simulink model "REFvsFI_ML2017a"  (R2017a)
settings: Solver=FixedStepAuto  StartTime=0.0  StopTime=T  RelTol=1e-3  EnableMultiTasking=on
values from neighbouring files (symbols this model uses):
  Ts = 1    [TestDataGen.m]
libraries: My_FI_Operations x114, simulink x2
(part 1 of 2)
settings Model: FPTShortcutValueString='{{},{''BaselineRun'',1,1,1,''BaselineRun'','''',{},''M'',''D'',''''}}'  OrderedModelArguments=off  Creator=kavru  LastModifiedBy=kolbe
settings DataIOCC: ReturnWorkspaceOutputs=on
settings OptimizationCC: BlockReduction=off  ConditionallyExecuteInputs=off
settings DebuggingCC: SignalRangeChecking=warning  SingleTaskRateTransMsg=error
settings SFSimCC: SimUseLocalCustomCode=on
settings RTWCC: RTWUseLocalCustomCode=on

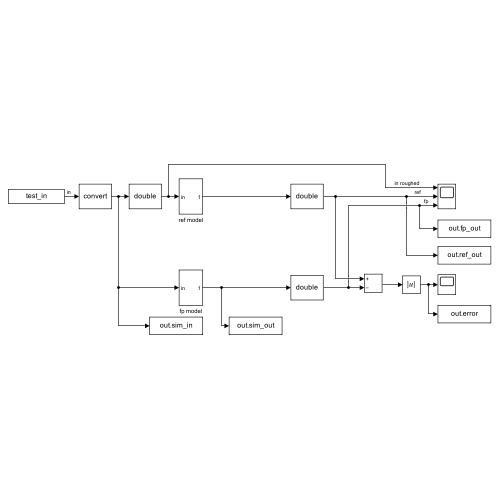
[thumbnail: Simulink's stored preview of the top-level diagram]
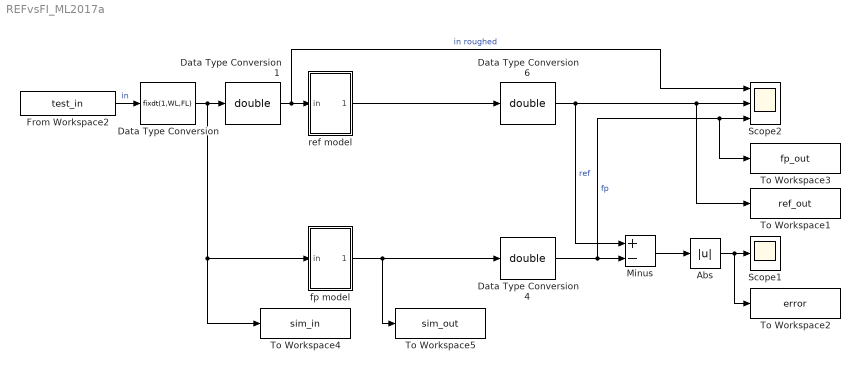
== system REFvsFI_ML2017a ==
  Abs : Abs
  Data Type Conversion : DataTypeConversion  OutDataTypeStr=fixdt(1,WL,FL)  RndMeth=Nearest  SaturateOnIntegerOverflow=on
  Data Type Conversion1 : DataTypeConversion  OutDataTypeStr=double  RndMeth=Nearest
  Data Type Conversion4 : DataTypeConversion  OutDataTypeStr=double  RndMeth=Nearest
  Data Type Conversion6 : DataTypeConversion  OutDataTypeStr=double  RndMeth=Nearest
  From Workspace2 : FromWorkspace  VariableName=test_in  OutDataTypeStr=double  SampleTime=Ts
  Minus : Sum  Inputs=+-
  Scope1 : Scope
  Scope2 : Scope  NumInputPorts=3
  To Workspace1 : ToWorkspace  VariableName=ref_out  SaveFormat=Timeseries  SampleTime=-1
  To Workspace2 : ToWorkspace  VariableName=error  SaveFormat=Timeseries  SampleTime=-1
  To Workspace3 : ToWorkspace  VariableName=fp_out  SaveFormat=Timeseries  SampleTime=-1
  To Workspace4 : ToWorkspace  VariableName=sim_in  SaveFormat=Timeseries  SampleTime=-1
  To Workspace5 : ToWorkspace  VariableName=sim_out  SaveFormat=Timeseries  SampleTime=-1
  fp model : Subsystem
  ref model : Subsystem
  wires:
  From Workspace2/1 -> Data Type Conversion/1  "in"
  Minus/1 -> Abs/1
  Abs/1 -> Scope1/1, To Workspace2/1
  fp model/1(Out1) -> To Workspace5/1, Data Type Conversion4/1
  Data Type Conversion4/1 -> Minus/2, To Workspace3/1, Scope2/3  "fp"
  Data Type Conversion6/1 -> Scope2/2, To Workspace1/1, Minus/1  "ref"
  Data Type Conversion1/1 -> Scope2/1, ref model/1(in)  "in roughed"
  Data Type Conversion/1 -> To Workspace4/1, fp model/1(in), Data Type Conversion1/1
  ref model/1(Out1) -> Data Type Conversion6/1

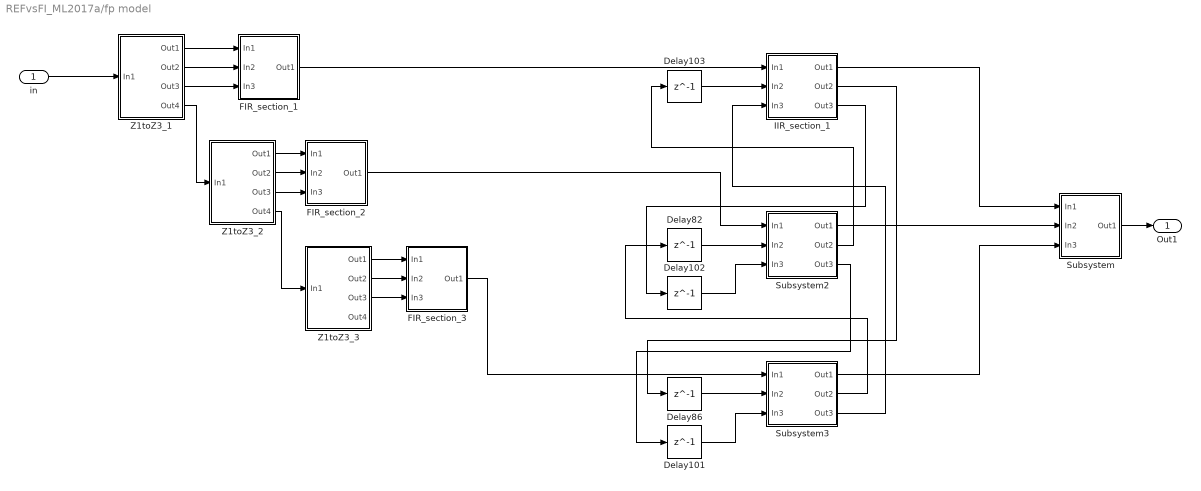
== system REFvsFI_ML2017a/fp model ==
  in : Inport
  Delay{82,86,101..103} (5 alike) : Delay  DelayLength=1  SampleTime=3*Ts
  FIR_section_1 : Subsystem
  FIR_section_2 : Subsystem
  FIR_section_3 : Subsystem
  IIR_section_1 : Subsystem
  Subsystem : Subsystem
  Subsystem2 : Subsystem
  Subsystem3 : Subsystem
  Z1toZ3_1 : Subsystem
  Z1toZ3_2 : Subsystem
  Z1toZ3_3 : Subsystem
  Out1 : Outport
  wires:
  in/1 -> Z1toZ3_1/1(In1)
  Z1toZ3_1/4(Out4) -> Z1toZ3_2/1(In1)
  Z1toZ3_2/4(Out4) -> Z1toZ3_3/1(In1)
  Z1toZ3_1/1(Out1) -> FIR_section_1/1(In1)
  Z1toZ3_1/2(Out2) -> FIR_section_1/2(In2)
  Z1toZ3_1/3(Out3) -> FIR_section_1/3(In3)
  Z1toZ3_2/1(Out1) -> FIR_section_2/1(In1)
  Z1toZ3_2/2(Out2) -> FIR_section_2/2(In2)
  Z1toZ3_2/3(Out3) -> FIR_section_2/3(In3)
  Z1toZ3_3/1(Out1) -> FIR_section_3/1(In1)
  Z1toZ3_3/2(Out2) -> FIR_section_3/2(In2)
  Z1toZ3_3/3(Out3) -> FIR_section_3/3(In3)
  Subsystem/1(Out1) -> Out1/1
  FIR_section_1/1(Out1) -> IIR_section_1/1(In1)
  Delay103/1 -> IIR_section_1/2(In2)
  IIR_section_1/2(Out2) -> Delay86/1
  IIR_section_1/1(Out1) -> Subsystem/1(In1)
  IIR_section_1/3(Out3) -> Delay102/1
  FIR_section_2/1(Out1) -> Subsystem2/1(In1)
  Delay102/1 -> Subsystem2/3(In3)
  Delay82/1 -> Subsystem2/2(In2)
  Subsystem2/1(Out1) -> Subsystem/2(In2)
  Subsystem2/2(Out2) -> Delay103/1
  Subsystem2/3(Out3) -> Delay101/1
  Delay86/1 -> Subsystem3/2(In2)
  Delay101/1 -> Subsystem3/3(In3)
  FIR_section_3/1(Out1) -> Subsystem3/1(In1)
  Subsystem3/3(Out3) -> IIR_section_1/3(In3)
  Subsystem3/1(Out1) -> Subsystem/3(In3)
  Subsystem3/2(Out2) -> Delay82/1

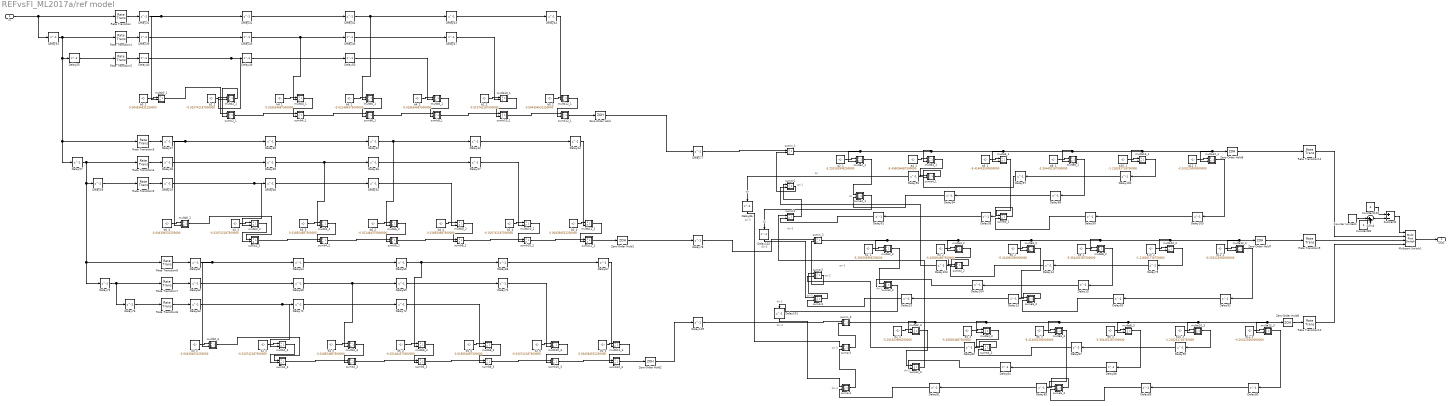
== system REFvsFI_ML2017a/ref model ==
  note: dn-1
  note: dn-2
  note: qn-3
  note: dn-3
  note: qn
  note: dn
  note: dn-4
  note: dn-2
  note: dn-1
  note: qn
  note: dn-4
  note: dn
  note: dn-3
  note: qn-2
  note: qn-3
  note: qn-1
  note: qn-1
  in : Inport
  Constant102 : Constant  Value=4
  Constant82 : Constant
  Counter Limited1 : simulink/Sources/Counter Limited  uplimit=2  tsamp=Ts
  Delay{13..15,23,27..37,39..50,52,60..72,75,77..78,80..82,84..95,97..105,109} (69 alike) : Delay  DelayLength=1  SampleTime=3*Ts
  Delay{53,55,57,59,74,76} (6 alike) : Delay  DelayLength=1  SampleTime=Ts
  Multiport Switch1 : MultiPortSwitch  OutDataTypeStr=double  RndMeth=Nearest
  Rate Transition{,1..8} (9 alike) : RateTransition  OutPortSampleTime=3*Ts
  Rate Transition10 : RateTransition  OutPortSampleTime=Ts
  Rate Transition12 : RateTransition  OutPortSampleTime=Ts
  Rate Transition9 : RateTransition  OutPortSampleTime=Ts
  Subtract2 : Sum  Inputs=+-
  Sum4 : Sum  Inputs=|++
  Zero-Order Hold{,1..2,6..8} (6 alike) : ZeroOrderHold  SampleTime=3*Ts
  a10_1 : Constant  Value=-1.218261718750000  OutDataTypeStr=double
  a10_2 : Constant  Value=-1.218261718750000  OutDataTypeStr=double
  a10_3 : Constant  Value=-1.218261718750000  OutDataTypeStr=double
  a12_1 : Constant  Value=-0.203125000000000  OutDataTypeStr=double
  a12_2 : Constant  Value=-0.203125000000000  OutDataTypeStr=double
  a12_3 : Constant  Value=-0.203125000000000  OutDataTypeStr=double
  a2_1 : Constant  Value=-3.291503906250000  OutDataTypeStr=double
  a2_2 : Constant  Value=-3.291503906250000  OutDataTypeStr=double
  a2_3 : Constant  Value=-3.291503906250000  OutDataTypeStr=double
  a4_1 : Constant  Value=-5.456054687500000  OutDataTypeStr=double
  a4_2 : Constant  Value=-5.456054687500000  OutDataTypeStr=double
  a4_3 : Constant  Value=-5.456054687500000  OutDataTypeStr=double
  a6_1 : Constant  Value=-5.414062500000000  OutDataTypeStr=double
  a6_2 : Constant  Value=-5.414062500000000  OutDataTypeStr=double
  a6_3 : Constant  Value=-5.414062500000000  OutDataTypeStr=double
  a8_1 : Constant  Value=-3.354492187500000  OutDataTypeStr=double
  a8_2 : Constant  Value=-3.354492187500000  OutDataTypeStr=double
  a8_3 : Constant  Value=-3.354492187500000  OutDataTypeStr=double
  b0_{1..6} (6 alike) : Constant  Value=0.004394531250000  OutDataTypeStr=double
  b2_{1..6} (6 alike) : Constant  Value=-0.010742187500000  OutDataTypeStr=double
  b4_{1..6} (6 alike) : Constant  Value=0.018554687500000  OutDataTypeStr=double
  b6_1 : Constant  Value=-0.021484375000000  OutDataTypeStr=double
  b6_2 : Constant  Value=-0.021484375000000  OutDataTypeStr=double
  b6_3 : Constant  Value=-0.021484375000000  OutDataTypeStr=double
  multa10_1 : Subsystem  AncestorBlock=My_FI_Operations/multa10_
      mask Display: disp('x')
  multa10_2 : Subsystem  AncestorBlock=My_FI_Operations/multa10_
      mask Display: disp('x')
  multa10_3 : Subsystem  AncestorBlock=My_FI_Operations/multa10_
      mask Display: disp('x')
  multa12_1 : Subsystem  AncestorBlock=My_FI_Operations/multa12_
      mask Display: disp('x')
  multa12_2 : Subsystem  AncestorBlock=My_FI_Operations/multa12_
      mask Display: disp('x')
  multa12_3 : Subsystem  AncestorBlock=My_FI_Operations/multa12_
      mask Display: disp('x')
  multa2_1 : Subsystem  AncestorBlock=My_FI_Operations/multa2_
      mask Display: disp('x')
  multa2_2 : Subsystem  AncestorBlock=My_FI_Operations/multa2_
      mask Display: disp('x')
  multa2_3 : Subsystem  AncestorBlock=My_FI_Operations/multa2_
      mask Display: disp('x')
  multa4_1 : Subsystem  AncestorBlock=My_FI_Operations/multa4_
      mask Display: disp('x')
  multa4_2 : Subsystem  AncestorBlock=My_FI_Operations/multa4_
      mask Display: disp('x')
  multa4_3 : Subsystem  AncestorBlock=My_FI_Operations/multa4_
      mask Display: disp('x')
  multa6_1 : Subsystem  AncestorBlock=My_FI_Operations/multa6_
      mask Display: disp('x')
  multa6_2 : Subsystem  AncestorBlock=My_FI_Operations/multa6_
      mask Display: disp('x')
  multa6_3 : Subsystem  AncestorBlock=My_FI_Operations/multa6_
      mask Display: disp('x')
  multa8_1 : Subsystem  AncestorBlock=My_FI_Operations/multa8_
      mask Display: disp('x')
  multa8_2 : Subsystem  AncestorBlock=My_FI_Operations/multa8_
      mask Display: disp('x')
  multa8_3 : Subsystem  AncestorBlock=My_FI_Operations/multa8_
      mask Display: disp('x')
  multb0_1 : Subsystem  AncestorBlock=My_FI_Operations/multb0_
      mask Display: disp('x')
  multb0_2 : Subsystem  AncestorBlock=My_FI_Operations/multb0_
      mask Display: disp('x')
  multb0_3 : Subsystem  AncestorBlock=My_FI_Operations/multb0_
      mask Display: disp('x')
  multb10_1 : Subsystem  AncestorBlock=My_FI_Operations/multb10_
      mask Display: disp('x')
  multb10_2 : Subsystem  AncestorBlock=My_FI_Operations/multb10_
      mask Display: disp('x')
  multb10_3 : Subsystem  AncestorBlock=My_FI_Operations/multb10_
      mask Display: disp('x')
  multb12_1 : Subsystem  AncestorBlock=My_FI_Operations/multb12_
      mask Display: disp('x')
  multb12_2 : Subsystem  AncestorBlock=My_FI_Operations/multb12_
      mask Display: disp('x')
  multb12_3 : Subsystem  AncestorBlock=My_FI_Operations/multb12_
      mask Display: disp('x')
  multb2_1 : Subsystem  AncestorBlock=My_FI_Operations/multb2_
      mask Display: disp('x')
  multb2_2 : Subsystem  AncestorBlock=My_FI_Operations/multb2_
      mask Display: disp('x')
  multb2_3 : Subsystem  AncestorBlock=My_FI_Operations/multb2_
      mask Display: disp('x')
  multb4_1 : Subsystem  AncestorBlock=My_FI_Operations/multb4_
      mask Display: disp('x')
  multb4_2 : Subsystem  AncestorBlock=My_FI_Operations/multb4_
      mask Display: disp('x')
  multb4_3 : Subsystem  AncestorBlock=My_FI_Operations/multb4_
      mask Display: disp('x')
  multb6_1 : Subsystem  AncestorBlock=My_FI_Operations/multb6_
      mask Display: disp('x')
  multb6_2 : Subsystem  AncestorBlock=My_FI_Operations/multb6_
      mask Display: disp('x')
  multb6_3 : Subsystem  AncestorBlock=My_FI_Operations/multb6_
      mask Display: disp('x')
  multb8_1 : Subsystem  AncestorBlock=My_FI_Operations/multb8_
      mask Display: disp('x')
  multb8_2 : Subsystem  AncestorBlock=My_FI_Operations/multb8_
      mask Display: disp('x')
  multb8_3 : Subsystem  AncestorBlock=My_FI_Operations/multb8_
      mask Display: disp('x')
  suma2_1 : Subsystem  AncestorBlock=My_FI_Operations/suma2_
      mask Display: disp('+')
  suma2_2 : Subsystem  AncestorBlock=My_FI_Operations/suma2_
      mask Display: disp('+')
  suma2_3 : Subsystem  AncestorBlock=My_FI_Operations/suma2_
      mask Display: disp('+')
  suma4_1 : Subsystem  AncestorBlock=My_FI_Operations/suma4_
      mask Display: disp('+')
  suma4_2 : Subsystem  AncestorBlock=My_FI_Operations/suma4_
      mask Display: disp('+')
  suma4_3 : Subsystem  AncestorBlock=My_FI_Operations/suma4_
      mask Display: disp('+')
  suma6_1 : Subsystem  AncestorBlock=My_FI_Operations/suma6_
      mask Display: disp('+')
  suma6_2 : Subsystem  AncestorBlock=My_FI_Operations/suma6_
      mask Display: disp('+')
  suma6_3 : Subsystem  AncestorBlock=My_FI_Operations/suma6_
      mask Display: disp('+')
  sumb10_1 : Subsystem  AncestorBlock=My_FI_Operations/sumb10_
      mask Display: disp('+')
  sumb10_2 : Subsystem  AncestorBlock=My_FI_Operations/sumb10_
      mask Display: disp('+')
  sumb10_3 : Subsystem  AncestorBlock=My_FI_Operations/sumb10_
      mask Display: disp('+')
  sumb12_1 : Subsystem  AncestorBlock=My_FI_Operations/sumb12_
      mask Display: disp('+')
  sumb12_2 : Subsystem  AncestorBlock=My_FI_Operations/sumb12_
      mask Display: disp('+')
  sumb12_3 : Subsystem  AncestorBlock=My_FI_Operations/sumb12_
      mask Display: disp('+')
  sumb2_1 : Subsystem  AncestorBlock=My_FI_Operations/sumb2_
      mask Display: disp('+')
  sumb2_2 : Subsystem  AncestorBlock=My_FI_Operations/sumb2_
      mask Display: disp('+')
  sumb2_3 : Subsystem  AncestorBlock=My_FI_Operations/sumb2_
      mask Display: disp('+')
  sumb4_1 : Subsystem  AncestorBlock=My_FI_Operations/sumb4_
      mask Display: disp('+')
  sumb4_2 : Subsystem  AncestorBlock=My_FI_Operations/sumb4_
      mask Display: disp('+')
  sumb4_3 : Subsystem  AncestorBlock=My_FI_Operations/sumb4_
      mask Display: disp('+')
  sumb6_1 : Subsystem  AncestorBlock=My_FI_Operations/sumb6_
      mask Display: disp('+')
  sumb6_2 : Subsystem  AncestorBlock=My_FI_Operations/sumb6_
      mask Display: disp('+')
  sumb6_3 : Subsystem  AncestorBlock=My_FI_Operations/sumb6_
      mask Display: disp('+')
  sumb8_1 : Subsystem  AncestorBlock=My_FI_Operations/sumb8_
      mask Display: disp('+')
  sumb8_2 : Subsystem  AncestorBlock=My_FI_Operations/sumb8_
      mask Display: disp('+')
  sumb8_3 : Subsystem  AncestorBlock=My_FI_Operations/sumb8_
      mask Display: disp('+')
  sumd-2 : Subsystem  AncestorBlock=My_FI_Operations/sumd-2
      mask Display: disp('+')
  sumd-3 : Subsystem  AncestorBlock=My_FI_Operations/sumd-3
      mask Display: disp('+')
  sumd-4 : Subsystem  AncestorBlock=My_FI_Operations/sumd-4
      mask Display: disp('+')
  sumin_1 : Subsystem  AncestorBlock=My_FI_Operations/sumin_
      mask Display: disp('+')
  sumin_2 : Subsystem  AncestorBlock=My_FI_Operations/sumin_
      mask Display: disp('+')
  sumin_3 : Subsystem  AncestorBlock=My_FI_Operations/sumin_
      mask Display: disp('+')
  sumq-1 : Subsystem  AncestorBlock=My_FI_Operations/sumq-1
      mask Display: disp('+')
  sumq-2 : Subsystem  AncestorBlock=My_FI_Operations/sumq-2
      mask Display: disp('+')
  sumq-3 : Subsystem  AncestorBlock=My_FI_Operations/sumq-3
      mask Display: disp('+')
  Out1 : Outport
  wires:
  Delay77/1 -> sumin_1/1(In1)
  Delay42/1 -> multb6_1/2(In1), Delay43/1
  multb6_2/1(Out1) -> sumb6_2/2(In1)
  Delay53/1 -> Rate Transition1/1, Rate Transition3/1, Delay57/1, Delay55/1
  Delay78/1 -> sumin_2/1(In1)
  sumin_2/1(Out1) -> multa2_2/2(In1), multa4_2/2(In1), multa6_2/2(In1), multa8_2/2(In1), multa10_2/2(In1), multa12_2/2(In1), Zero-Order Hold7/1
  b0_6/1 -> multb12_3/1(In2)
  Delay69/1 -> Delay70/1
  Delay101/1 -> sumd-4/1(In1)
  Delay31/1 -> multb0_1/2(In1), Delay41/1
  sumq-2/1(Out1) -> sumin_2/2(In2)
  Delay32/1 -> multb6_2/2(In1), Delay33/1
  multa8_3/1(Out1) -> Delay88/1
  multb6_1/1(Out1) -> sumb6_1/2(In1)
  Delay94/1 -> suma2_1/2(In1)
  Delay68/1 -> multb4_3/2(In1), Delay69/1
  Delay41/1 -> Delay42/1
  Delay85/1 -> Delay81/1
  Zero-Order Hold/1 -> Delay77/1
  Delay64/1 -> Delay65/1
  b2_4/1 -> multb10_2/1(In2)
  sumin_1/1(Out1) -> multa2_1/2(In1), multa4_1/2(In1), multa6_1/2(In1), multa8_1/2(In1), multa10_1/2(In1), multa12_1/2(In1), Zero-Order Hold6/1
  sumb4_3/1(Out1) -> sumb6_3/1(In2)
  b4_5/1 -> multb4_3/1(In2)
  Zero-Order Hold2/1 -> Delay109/1
  Zero-Order Hold1/1 -> Delay78/1
  Delay84/1 -> suma2_3/2(In1)
  Delay27/1 -> multb0_2/2(In1), Delay30/1
  in/1 -> Delay53/1, Rate Transition/1
  Delay100/1 -> Delay97/1
  multa2_3/1(Out1) -> suma2_3/1(In2)
  Delay65/1 -> multb6_3/2(In1), Delay66/1
  Delay28/1 -> Delay35/1
  Delay33/1 -> Delay34/1
  Delay57/1 -> Rate Transition4/1, Rate Transition6/1, Delay74/1, Delay59/1
  Delay48/1 -> Delay52/1
  Delay98/1 -> Delay94/1
  multa10_2/1(Out1) -> Delay75/1
  Delay40/1 -> multb2_1/2(In1), Delay49/1
  Delay13/1 -> Delay23/1
  a10_2/1 -> multa10_2/1(In2)
  sumb2_3/1(Out1) -> sumb4_3/1(In2)
  a4_3/1 -> multa4_3/1(In2)
  sumd-3/1(Out1) -> sumq-2/1(In1)
  suma6_3/1(Out1) -> Delay85/1
  sumb12_1/1(Out1) -> Zero-Order Hold/1
  Delay63/1 -> multb2_3/2(In1), Delay71/1
  Multiport Switch1/1 -> Out1/1
  a12_1/1 -> multa12_1/1(In2)
  multb4_3/1(Out1) -> sumb4_3/2(In1)
  multa8_2/1(Out1) -> Delay15/1
  sumq-3/1(Out1) -> sumin_3/2(In2)
  Constant82/1 -> Sum4/2
  Delay15/1 -> Delay104/1
  Delay109/1 -> sumin_3/1(In1)
  Delay86/1 -> sumq-3/1(In1)
  multa4_2/1(Out1) -> suma4_2/1(In1)
  sumd-4/1(Out1) -> sumq-3/2(In2)
  b0_1/1 -> multb0_1/1(In2)
  Delay88/1 -> Delay84/1
  multa6_3/1(Out1) -> suma6_3/1(In1)
  Counter Limited1/1 -> Sum4/1
  sumb6_2/1(Out1) -> sumb8_2/1(In2)
  sumb8_3/1(Out1) -> sumb10_3/1(In2)
  Delay61/1 -> multb0_3/2(In1), Delay64/1
  Delay91/1 -> sumd-2/2(In2)
  multa4_3/1(Out1) -> suma4_3/1(In1)
  a2_3/1 -> multa2_3/1(In2)
  a10_3/1 -> multa10_3/1(In2)
  a12_3/1 -> multa12_3/1(In2)
  b0_2/1 -> multb12_1/1(In2)
  a12_2/1 -> multa12_2/1(In2)
  Delay95/1 -> Delay91/1
  multb12_1/1(Out1) -> sumb12_1/2(In1)
  b2_2/1 -> multb10_1/1(In2)
  a6_3/1 -> multa6_3/1(In2)
  sumin_3/1(Out1) -> multa2_3/2(In1), multa4_3/2(In1), multa6_3/2(In1), multa8_3/2(In1), multa10_3/2(In1), multa12_3/2(In1), Zero-Order Hold8/1
  Delay62/1 -> Delay68/1
  Delay70/1 -> multb10_3/2(In1)
  a4_1/1 -> multa4_1/1(In2)
  Delay74/1 -> Rate Transition7/1, Delay76/1
  Delay50/1 -> multb8_1/2(In1)
  sumd-2/1(Out1) -> sumq-1/1(In2)
  a2_1/1 -> multa2_1/1(In2)
  sumb8_1/1(Out1) -> sumb10_1/1(In2)
  Delay14/1 -> suma4_2/2(In2)
  Delay87/1 -> suma4_3/2(In2)
  a4_2/1 -> multa4_2/1(In2)
  Zero-Order Hold6/1 -> Rate Transition12/1
  Subtract2/1 -> Multiport Switch1/1
  a6_2/1 -> multa6_2/1(In2)
  multb2_3/1(Out1) -> sumb2_3/2(In1)
  multb4_1/1(Out1) -> sumb4_1/2(In1)
  Delay81/1 -> sumd-4/2(In2)
  Delay89/1 -> suma6_3/2(In2)
  Delay35/1 -> multb4_2/2(In1), Delay36/1
  Delay34/1 -> multb12_2/2(In1)
  multb2_1/1(Out1) -> sumb2_1/2(In1)
  multb6_3/1(Out1) -> sumb6_3/2(In1)
  a8_1/1 -> multa8_1/1(In2)
  Delay52/1 -> multb8_2/2(In1)
  sumq-1/1(Out1) -> sumin_1/2(In2)
  b6_3/1 -> multb6_3/1(In2)
  sumb10_3/1(Out1) -> sumb12_3/1(In2)
  multb8_3/1(Out1) -> sumb8_3/2(In1)
  a2_2/1 -> multa2_2/1(In2)
  Delay55/1 -> Rate Transition2/1
  Delay93/1 -> Delay86/1
  multa10_3/1(Out1) -> Delay90/1
  multb10_3/1(Out1) -> sumb10_3/2(In1)
  Delay60/1 -> suma6_2/2(In2)
  suma2_3/1(Out1) -> sumd-2/1(In1)
  Delay30/1 -> Delay32/1
  sumb4_1/1(Out1) -> sumb6_1/1(In2)
  multb2_2/1(Out1) -> sumb2_2/2(In1)
  b2_1/1 -> multb2_1/1(In2)
  Delay23/1 -> sumd-3/2(In2)
  b4_1/1 -> multb4_1/1(In2)
  multb10_1/1(Out1) -> sumb10_1/2(In1)
  Delay47/1 -> multb10_1/2(In1)
  Delay103/1 -> sumq-1/2(In1)
  Constant102/1 -> Subtract2/1
  Delay36/1 -> Delay37/1
  sumb10_1/1(Out1) -> sumb12_1/1(In2)
  b6_2/1 -> multb6_2/1(In2)
  b6_1/1 -> multb6_1/1(In2)
  b0_4/1 -> multb12_2/1(In2)
  multb8_1/1(Out1) -> sumb8_1/2(In1)
  Delay29/1 -> multb2_2/2(In1), Delay48/1
  b4_2/1 -> multb8_1/1(In2)
  Delay59/1 -> Rate Transition5/1
  b2_6/1 -> multb10_3/1(In2)
  sumb2_2/1(Out1) -> sumb4_2/1(In2)
  multb4_2/1(Out1) -> sumb4_2/2(In1)
  Delay71/1 -> Delay72/1
  multb0_2/1(Out1) -> sumb2_2/1(In2)
  sumb4_2/1(Out1) -> sumb6_2/1(In2)
  multb8_2/1(Out1) -> sumb8_2/2(In1)
  multb12_2/1(Out1) -> sumb12_2/2(In1)
  sumb8_2/1(Out1) -> sumb10_2/1(In2)
  multb10_2/1(Out1) -> sumb10_2/2(In1)
  b0_3/1 -> multb0_2/1(In2)
  suma2_1/1(Out1) -> Delay102/1
  b2_3/1 -> multb2_2/1(In2)
  Delay39/1 -> Delay45/1
  b4_6/1 -> multb8_3/1(In2)
  Delay66/1 -> Delay67/1
  multb12_3/1(Out1) -> sumb12_3/2(In1)
  sumb6_3/1(Out1) -> sumb8_3/1(In2)
  Delay67/1 -> multb12_3/2(In1)
  suma2_2/1(Out1) -> Delay101/1
  suma4_3/1(Out1) -> Delay82/1
  multa6_2/1(Out1) -> suma6_2/1(In1)
  suma4_2/1(Out1) -> Delay103/1
  Delay104/1 -> suma2_2/2(In1)
  Delay99/1 -> suma6_1/2(In2)
  Delay80/1 -> Delay89/1
  sumb2_1/1(Out1) -> sumb4_1/1(In2)
  multa12_1/1(Out1) -> Delay105/1
  a10_1/1 -> multa10_1/1(In2)
  multa10_1/1(Out1) -> Delay100/1
  Delay44/1 -> multb12_1/2(In1)
  Delay82/1 -> sumq-2/2(In2)
  multa12_3/1(Out1) -> Delay80/1
  Delay90/1 -> Delay87/1
  Delay75/1 -> Delay14/1
  Zero-Order Hold7/1 -> Rate Transition9/1
  suma6_1/1(Out1) -> Delay95/1
  Zero-Order Hold8/1 -> Rate Transition10/1
  sumb10_2/1(Out1) -> sumb12_2/1(In2)
  sumb12_2/1(Out1) -> Zero-Order Hold1/1
  multb0_3/1(Out1) -> sumb2_3/1(In2)
  multa12_2/1(Out1) -> Delay92/1
  Delay105/1 -> Delay99/1
  Delay45/1 -> multb4_1/2(In1), Delay46/1
  multa2_1/1(Out1) -> suma2_1/1(In2)
  multa4_1/1(Out1) -> suma4_1/1(In1)
  Delay102/1 -> sumd-3/1(In1)
  Delay92/1 -> Delay60/1
  a8_2/1 -> multa8_2/1(In2)
  b0_5/1 -> multb0_3/1(In2)
  Delay72/1 -> multb8_3/2(In1)
  Delay97/1 -> suma4_1/2(In2)
  b4_4/1 -> multb8_2/1(In2)
  multa6_1/1(Out1) -> suma6_1/1(In1)
  sumb12_3/1(Out1) -> Zero-Order Hold2/1
  suma6_2/1(Out1) -> Delay13/1
  a6_1/1 -> multa6_1/1(In2)
  Delay37/1 -> multb10_2/2(In1)
  Delay43/1 -> Delay44/1
  multa2_2/1(Out1) -> suma2_2/1(In2)
  Sum4/1 -> Subtract2/2
  multa8_1/1(Out1) -> Delay98/1
  Delay76/1 -> Rate Transition8/1
  suma4_1/1(Out1) -> Delay93/1
  multb0_1/1(Out1) -> sumb2_1/1(In2)
  b4_3/1 -> multb4_2/1(In2)
  b2_5/1 -> multb2_3/1(In2)
  a8_3/1 -> multa8_3/1(In2)
  Delay46/1 -> Delay47/1
  sumb6_1/1(Out1) -> sumb8_1/1(In2)
  Delay49/1 -> Delay50/1
  Rate Transition/1 -> Delay31/1
  Rate Transition1/1 -> Delay39/1
  Rate Transition2/1 -> Delay40/1
  Rate Transition3/1 -> Delay27/1
  Rate Transition4/1 -> Delay28/1
  Rate Transition5/1 -> Delay29/1
  Rate Transition6/1 -> Delay61/1
  Rate Transition7/1 -> Delay62/1
  Rate Transition8/1 -> Delay63/1
  Rate Transition12/1 -> Multiport Switch1/2
  Rate Transition9/1 -> Multiport Switch1/3
  Rate Transition10/1 -> Multiport Switch1/4

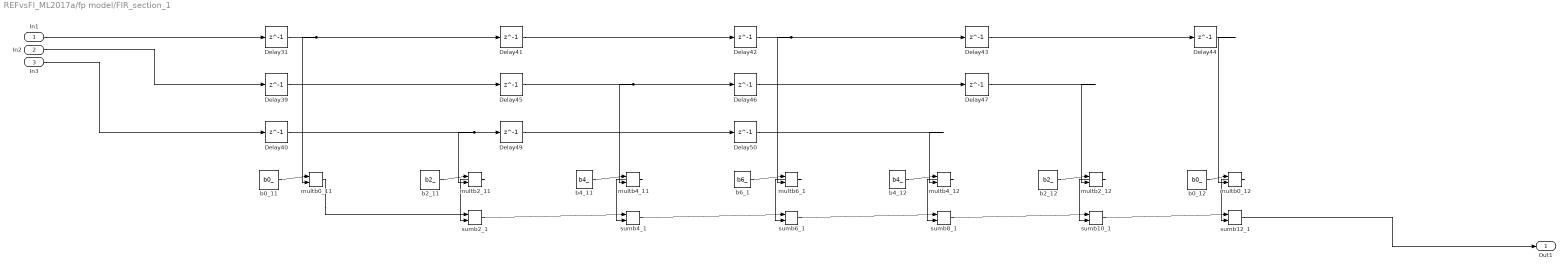
== system REFvsFI_ML2017a/fp model/FIR_section_1 ==
  In1 : Inport
  In2 : Inport  Port=2
  In3 : Inport  Port=3
  Delay{31,39..47,49..50} (12 alike) : Delay  DelayLength=1  SampleTime=3*Ts
  b0_11 : My_FI_Operations/b0_  SystemSampleTime=-1  Latency=0  AutoFrameSizeCalculation=off
  b0_12 : My_FI_Operations/b0_  SystemSampleTime=-1  Latency=0  AutoFrameSizeCalculation=off
  b2_11 : My_FI_Operations/b2_  SystemSampleTime=-1  Latency=0  AutoFrameSizeCalculation=off
  b2_12 : My_FI_Operations/b2_  SystemSampleTime=-1  Latency=0  AutoFrameSizeCalculation=off
  b4_11 : My_FI_Operations/b4_  SystemSampleTime=-1  Latency=0  AutoFrameSizeCalculation=off
  b4_12 : My_FI_Operations/b4_  SystemSampleTime=-1  Latency=0  AutoFrameSizeCalculation=off
  b6_1 : My_FI_Operations/b6_  SystemSampleTime=-1  Latency=0  AutoFrameSizeCalculation=off
  multb0_11 : My_FI_Operations/multb0_  SystemSampleTime=-1  Latency=0  AutoFrameSizeCalculation=off
  multb0_12 : My_FI_Operations/multb0_  SystemSampleTime=-1  Latency=0  AutoFrameSizeCalculation=off
  multb2_11 : My_FI_Operations/multb2_  SystemSampleTime=-1  Latency=0  AutoFrameSizeCalculation=off
  multb2_12 : My_FI_Operations/multb2_  SystemSampleTime=-1  Latency=0  AutoFrameSizeCalculation=off
  multb4_11 : My_FI_Operations/multb4_  SystemSampleTime=-1  Latency=0  AutoFrameSizeCalculation=off
  multb4_12 : My_FI_Operations/multb4_  SystemSampleTime=-1  Latency=0  AutoFrameSizeCalculation=off
  multb6_1 : My_FI_Operations/multb6_  SystemSampleTime=-1  Latency=0  AutoFrameSizeCalculation=off
  sumb10_1 : My_FI_Operations/sumb10_  SystemSampleTime=-1  Latency=0  AutoFrameSizeCalculation=off
  sumb12_1 : My_FI_Operations/sumb12_  SystemSampleTime=-1  Latency=0  AutoFrameSizeCalculation=off
  sumb2_1 : My_FI_Operations/sumb2_  SystemSampleTime=-1  Latency=0  AutoFrameSizeCalculation=off
  sumb4_1 : My_FI_Operations/sumb4_  SystemSampleTime=-1  Latency=0  AutoFrameSizeCalculation=off
  sumb6_1 : My_FI_Operations/sumb6_  SystemSampleTime=-1  Latency=0  AutoFrameSizeCalculation=off
  sumb8_1 : My_FI_Operations/sumb8_  SystemSampleTime=-1  Latency=0  AutoFrameSizeCalculation=off
  Out1 : Outport
  wires:
  In3/1 -> Delay40/1
  Delay39/1 -> Delay45/1
  Delay31/1 -> multb0_11/2, Delay41/1
  Delay47/1 -> multb2_12/2
  Delay49/1 -> Delay50/1
  b2_12/1 -> multb2_12/1
  Delay50/1 -> multb4_12/2
  sumb6_1/1 -> sumb8_1/1
  multb2_11/1 -> sumb2_1/2
  Delay46/1 -> Delay47/1
  b0_12/1 -> multb0_12/1
  b0_11/1 -> multb0_11/1
  b4_12/1 -> multb4_12/1
  sumb8_1/1 -> sumb10_1/1
  multb0_12/1 -> sumb12_1/2
  Delay45/1 -> multb4_11/2, Delay46/1
  Delay41/1 -> Delay42/1
  Delay42/1 -> multb6_1/2, Delay43/1
  sumb4_1/1 -> sumb6_1/1
  multb4_11/1 -> sumb4_1/2
  b6_1/1 -> multb6_1/1
  Delay44/1 -> multb0_12/2
  b2_11/1 -> multb2_11/1
  b4_11/1 -> multb4_11/1
  sumb12_1/1 -> Out1/1
  multb6_1/1 -> sumb6_1/2
  multb0_11/1 -> sumb2_1/1
  multb4_12/1 -> sumb8_1/2
  Delay40/1 -> multb2_11/2, Delay49/1
  sumb2_1/1 -> sumb4_1/1
  In2/1 -> Delay39/1
  multb2_12/1 -> sumb10_1/2
  Delay43/1 -> Delay44/1
  sumb10_1/1 -> sumb12_1/1
  In1/1 -> Delay31/1

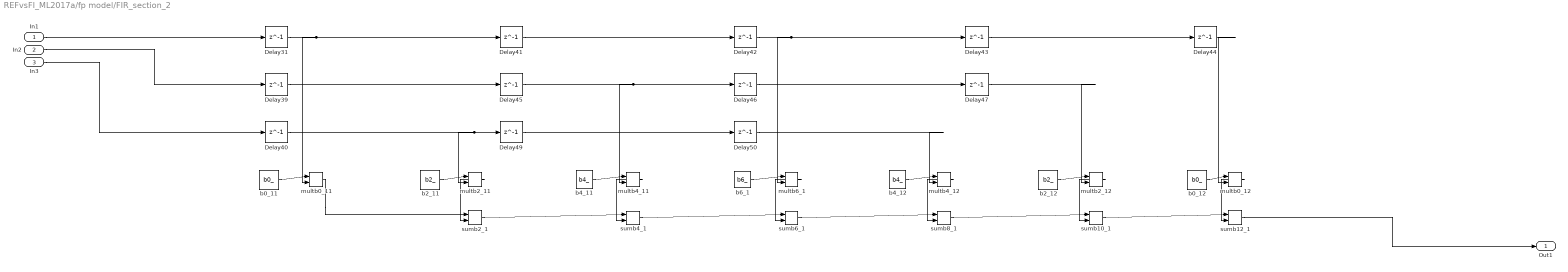
== system REFvsFI_ML2017a/fp model/FIR_section_2 ==
  In1 : Inport
  In2 : Inport  Port=2
  In3 : Inport  Port=3
  Delay{31,39..47,49..50} (12 alike) : Delay  DelayLength=1  SampleTime=3*Ts
  b0_11 : My_FI_Operations/b0_  SystemSampleTime=-1  Latency=0  AutoFrameSizeCalculation=off
  b0_12 : My_FI_Operations/b0_  SystemSampleTime=-1  Latency=0  AutoFrameSizeCalculation=off
  b2_11 : My_FI_Operations/b2_  SystemSampleTime=-1  Latency=0  AutoFrameSizeCalculation=off
  b2_12 : My_FI_Operations/b2_  SystemSampleTime=-1  Latency=0  AutoFrameSizeCalculation=off
  b4_11 : My_FI_Operations/b4_  SystemSampleTime=-1  Latency=0  AutoFrameSizeCalculation=off
  b4_12 : My_FI_Operations/b4_  SystemSampleTime=-1  Latency=0  AutoFrameSizeCalculation=off
  b6_1 : My_FI_Operations/b6_  SystemSampleTime=-1  Latency=0  AutoFrameSizeCalculation=off
  multb0_11 : My_FI_Operations/multb0_  SystemSampleTime=-1  Latency=0  AutoFrameSizeCalculation=off
  multb0_12 : My_FI_Operations/multb0_  SystemSampleTime=-1  Latency=0  AutoFrameSizeCalculation=off
  multb2_11 : My_FI_Operations/multb2_  SystemSampleTime=-1  Latency=0  AutoFrameSizeCalculation=off
  multb2_12 : My_FI_Operations/multb2_  SystemSampleTime=-1  Latency=0  AutoFrameSizeCalculation=off
  multb4_11 : My_FI_Operations/multb4_  SystemSampleTime=-1  Latency=0  AutoFrameSizeCalculation=off
  multb4_12 : My_FI_Operations/multb4_  SystemSampleTime=-1  Latency=0  AutoFrameSizeCalculation=off
  multb6_1 : My_FI_Operations/multb6_  SystemSampleTime=-1  Latency=0  AutoFrameSizeCalculation=off
  sumb10_1 : My_FI_Operations/sumb10_  SystemSampleTime=-1  Latency=0  AutoFrameSizeCalculation=off
  sumb12_1 : My_FI_Operations/sumb12_  SystemSampleTime=-1  Latency=0  AutoFrameSizeCalculation=off
  sumb2_1 : My_FI_Operations/sumb2_  SystemSampleTime=-1  Latency=0  AutoFrameSizeCalculation=off
  sumb4_1 : My_FI_Operations/sumb4_  SystemSampleTime=-1  Latency=0  AutoFrameSizeCalculation=off
  sumb6_1 : My_FI_Operations/sumb6_  SystemSampleTime=-1  Latency=0  AutoFrameSizeCalculation=off
  sumb8_1 : My_FI_Operations/sumb8_  SystemSampleTime=-1  Latency=0  AutoFrameSizeCalculation=off
  Out1 : Outport
  wires:
  In3/1 -> Delay40/1
  Delay39/1 -> Delay45/1
  Delay31/1 -> multb0_11/2, Delay41/1
  Delay47/1 -> multb2_12/2
  Delay49/1 -> Delay50/1
  b2_12/1 -> multb2_12/1
  Delay50/1 -> multb4_12/2
  sumb6_1/1 -> sumb8_1/1
  multb2_11/1 -> sumb2_1/2
  Delay46/1 -> Delay47/1
  b0_12/1 -> multb0_12/1
  b0_11/1 -> multb0_11/1
  b4_12/1 -> multb4_12/1
  sumb8_1/1 -> sumb10_1/1
  multb0_12/1 -> sumb12_1/2
  Delay45/1 -> multb4_11/2, Delay46/1
  Delay41/1 -> Delay42/1
  Delay42/1 -> multb6_1/2, Delay43/1
  sumb4_1/1 -> sumb6_1/1
  multb4_11/1 -> sumb4_1/2
  b6_1/1 -> multb6_1/1
  Delay44/1 -> multb0_12/2
  b2_11/1 -> multb2_11/1
  b4_11/1 -> multb4_11/1
  sumb12_1/1 -> Out1/1
  multb6_1/1 -> sumb6_1/2
  multb0_11/1 -> sumb2_1/1
  multb4_12/1 -> sumb8_1/2
  Delay40/1 -> multb2_11/2, Delay49/1
  sumb2_1/1 -> sumb4_1/1
  In2/1 -> Delay39/1
  multb2_12/1 -> sumb10_1/2
  Delay43/1 -> Delay44/1
  sumb10_1/1 -> sumb12_1/1
  In1/1 -> Delay31/1

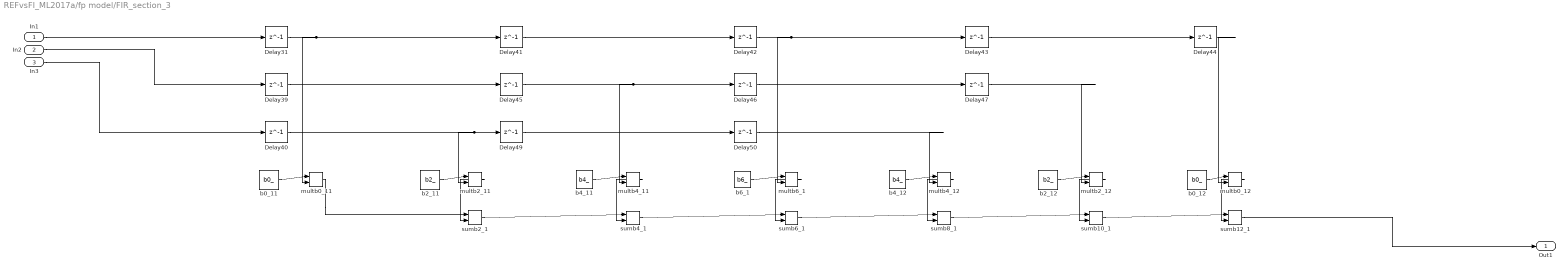
== system REFvsFI_ML2017a/fp model/FIR_section_3 ==
  In1 : Inport
  In2 : Inport  Port=2
  In3 : Inport  Port=3
  Delay{31,39..47,49..50} (12 alike) : Delay  DelayLength=1  SampleTime=3*Ts
  b0_11 : My_FI_Operations/b0_  SystemSampleTime=-1  Latency=0  AutoFrameSizeCalculation=off
  b0_12 : My_FI_Operations/b0_  SystemSampleTime=-1  Latency=0  AutoFrameSizeCalculation=off
  b2_11 : My_FI_Operations/b2_  SystemSampleTime=-1  Latency=0  AutoFrameSizeCalculation=off
  b2_12 : My_FI_Operations/b2_  SystemSampleTime=-1  Latency=0  AutoFrameSizeCalculation=off
  b4_11 : My_FI_Operations/b4_  SystemSampleTime=-1  Latency=0  AutoFrameSizeCalculation=off
  b4_12 : My_FI_Operations/b4_  SystemSampleTime=-1  Latency=0  AutoFrameSizeCalculation=off
  b6_1 : My_FI_Operations/b6_  SystemSampleTime=-1  Latency=0  AutoFrameSizeCalculation=off
  multb0_11 : My_FI_Operations/multb0_  SystemSampleTime=-1  Latency=0  AutoFrameSizeCalculation=off
  multb0_12 : My_FI_Operations/multb0_  SystemSampleTime=-1  Latency=0  AutoFrameSizeCalculation=off
  multb2_11 : My_FI_Operations/multb2_  SystemSampleTime=-1  Latency=0  AutoFrameSizeCalculation=off
  multb2_12 : My_FI_Operations/multb2_  SystemSampleTime=-1  Latency=0  AutoFrameSizeCalculation=off
  multb4_11 : My_FI_Operations/multb4_  SystemSampleTime=-1  Latency=0  AutoFrameSizeCalculation=off
  multb4_12 : My_FI_Operations/multb4_  SystemSampleTime=-1  Latency=0  AutoFrameSizeCalculation=off
  multb6_1 : My_FI_Operations/multb6_  SystemSampleTime=-1  Latency=0  AutoFrameSizeCalculation=off
  sumb10_1 : My_FI_Operations/sumb10_  SystemSampleTime=-1  Latency=0  AutoFrameSizeCalculation=off
  sumb12_1 : My_FI_Operations/sumb12_  SystemSampleTime=-1  Latency=0  AutoFrameSizeCalculation=off
  sumb2_1 : My_FI_Operations/sumb2_  SystemSampleTime=-1  Latency=0  AutoFrameSizeCalculation=off
  sumb4_1 : My_FI_Operations/sumb4_  SystemSampleTime=-1  Latency=0  AutoFrameSizeCalculation=off
  sumb6_1 : My_FI_Operations/sumb6_  SystemSampleTime=-1  Latency=0  AutoFrameSizeCalculation=off
  sumb8_1 : My_FI_Operations/sumb8_  SystemSampleTime=-1  Latency=0  AutoFrameSizeCalculation=off
  Out1 : Outport
  wires:
  In3/1 -> Delay40/1
  Delay39/1 -> Delay45/1
  Delay31/1 -> multb0_11/2, Delay41/1
  Delay47/1 -> multb2_12/2
  Delay49/1 -> Delay50/1
  b2_12/1 -> multb2_12/1
  Delay50/1 -> multb4_12/2
  sumb6_1/1 -> sumb8_1/1
  multb2_11/1 -> sumb2_1/2
  Delay46/1 -> Delay47/1
  b0_12/1 -> multb0_12/1
  b0_11/1 -> multb0_11/1
  b4_12/1 -> multb4_12/1
  sumb8_1/1 -> sumb10_1/1
  multb0_12/1 -> sumb12_1/2
  Delay45/1 -> multb4_11/2, Delay46/1
  Delay41/1 -> Delay42/1
  Delay42/1 -> multb6_1/2, Delay43/1
  sumb4_1/1 -> sumb6_1/1
  multb4_11/1 -> sumb4_1/2
  b6_1/1 -> multb6_1/1
  Delay44/1 -> multb0_12/2
  b2_11/1 -> multb2_11/1
  b4_11/1 -> multb4_11/1
  sumb12_1/1 -> Out1/1
  multb6_1/1 -> sumb6_1/2
  multb0_11/1 -> sumb2_1/1
  multb4_12/1 -> sumb8_1/2
  Delay40/1 -> multb2_11/2, Delay49/1
  sumb2_1/1 -> sumb4_1/1
  In2/1 -> Delay39/1
  multb2_12/1 -> sumb10_1/2
  Delay43/1 -> Delay44/1
  sumb10_1/1 -> sumb12_1/1
  In1/1 -> Delay31/1

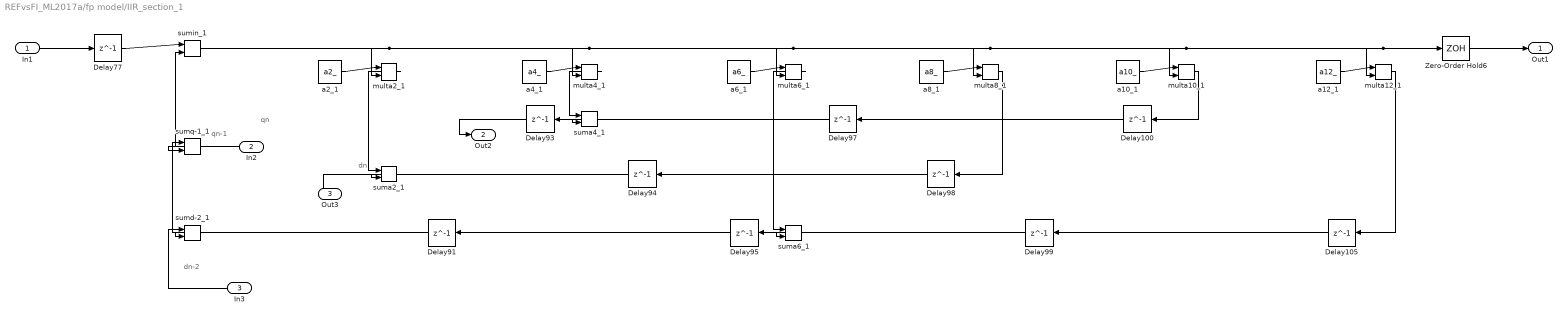
== system REFvsFI_ML2017a/fp model/IIR_section_1 ==
  note: dn
  note: dn-2
  note: qn
  note: qn-1
  In1 : Inport
  In2 : Inport  Port=2
  In3 : Inport  Port=3
  Delay{77,91,93..95,97..100,105} (10 alike) : Delay  DelayLength=1  SampleTime=3*Ts
  Zero-Order Hold6 : ZeroOrderHold  SampleTime=3*Ts
  a10_1 : My_FI_Operations/a10_  SystemSampleTime=-1  Latency=0  AutoFrameSizeCalculation=off
  a12_1 : My_FI_Operations/a12_  SystemSampleTime=-1  Latency=0  AutoFrameSizeCalculation=off
  a2_1 : My_FI_Operations/a2_  SystemSampleTime=-1  Latency=0  AutoFrameSizeCalculation=off
  a4_1 : My_FI_Operations/a4_  SystemSampleTime=-1  Latency=0  AutoFrameSizeCalculation=off
  a6_1 : My_FI_Operations/a6_  SystemSampleTime=-1  Latency=0  AutoFrameSizeCalculation=off
  a8_1 : My_FI_Operations/a8_  SystemSampleTime=-1  Latency=0  AutoFrameSizeCalculation=off
  multa10_1 : My_FI_Operations/multa10_  SystemSampleTime=-1  Latency=0  AutoFrameSizeCalculation=off
  multa12_1 : My_FI_Operations/multa12_  SystemSampleTime=-1  Latency=0  AutoFrameSizeCalculation=off
  multa2_1 : My_FI_Operations/multa2_  SystemSampleTime=-1  Latency=0  AutoFrameSizeCalculation=off
  multa4_1 : My_FI_Operations/multa4_  SystemSampleTime=-1  Latency=0  AutoFrameSizeCalculation=off
  multa6_1 : My_FI_Operations/multa6_  SystemSampleTime=-1  Latency=0  AutoFrameSizeCalculation=off
  multa8_1 : My_FI_Operations/multa8_  SystemSampleTime=-1  Latency=0  AutoFrameSizeCalculation=off
  suma2_1 : My_FI_Operations/suma2_  SystemSampleTime=-1  Latency=0  AutoFrameSizeCalculation=off
  suma4_1 : My_FI_Operations/suma4_  SystemSampleTime=-1  Latency=0  AutoFrameSizeCalculation=off
  suma6_1 : My_FI_Operations/suma6_  SystemSampleTime=-1  Latency=0  AutoFrameSizeCalculation=off
  sumd-2_1 : My_FI_Operations/sumd-2_  SystemSampleTime=-1  Latency=0  AutoFrameSizeCalculation=off
  sumin_1 : My_FI_Operations/sumin_  SystemSampleTime=-1  Latency=0  AutoFrameSizeCalculation=off
  sumq-1_1 : My_FI_Operations/sumq-1_  SystemSampleTime=-1  Latency=0  AutoFrameSizeCalculation=off
  Out1 : Outport
  Out2 : Outport  Port=2
  Out3 : Outport  Port=3
  wires:
  Delay77/1 -> sumin_1/1
  a12_1/1 -> multa12_1/1
  Delay98/1 -> Delay94/1
  Delay91/1 -> sumd-2_1/2
  sumin_1/1 -> multa2_1/2, multa4_1/2, multa6_1/2, multa8_1/2, multa10_1/2, multa12_1/2, Zero-Order Hold6/1
  Delay99/1 -> suma6_1/2
  Delay95/1 -> Delay91/1
  Delay94/1 -> suma2_1/2
  sumd-2_1/1 -> sumq-1_1/1
  a2_1/1 -> multa2_1/1
  multa4_1/1 -> suma4_1/1
  Delay100/1 -> Delay97/1
  Zero-Order Hold6/1 -> Out1/1
  multa6_1/1 -> suma6_1/1
  a10_1/1 -> multa10_1/1
  a4_1/1 -> multa4_1/1
  multa12_1/1 -> Delay105/1
  multa2_1/1 -> suma2_1/1
  Delay105/1 -> Delay99/1
  a8_1/1 -> multa8_1/1
  suma6_1/1 -> Delay95/1
  Delay97/1 -> suma4_1/2
  multa10_1/1 -> Delay100/1
  suma4_1/1 -> Delay93/1
  multa8_1/1 -> Delay98/1
  Delay93/1 -> Out2/1
  sumq-1_1/1 -> sumin_1/2
  a6_1/1 -> multa6_1/1
  In2/1 -> sumq-1_1/2
  In1/1 -> Delay77/1
  In3/1 -> sumd-2_1/1
  suma2_1/1 -> Out3/1

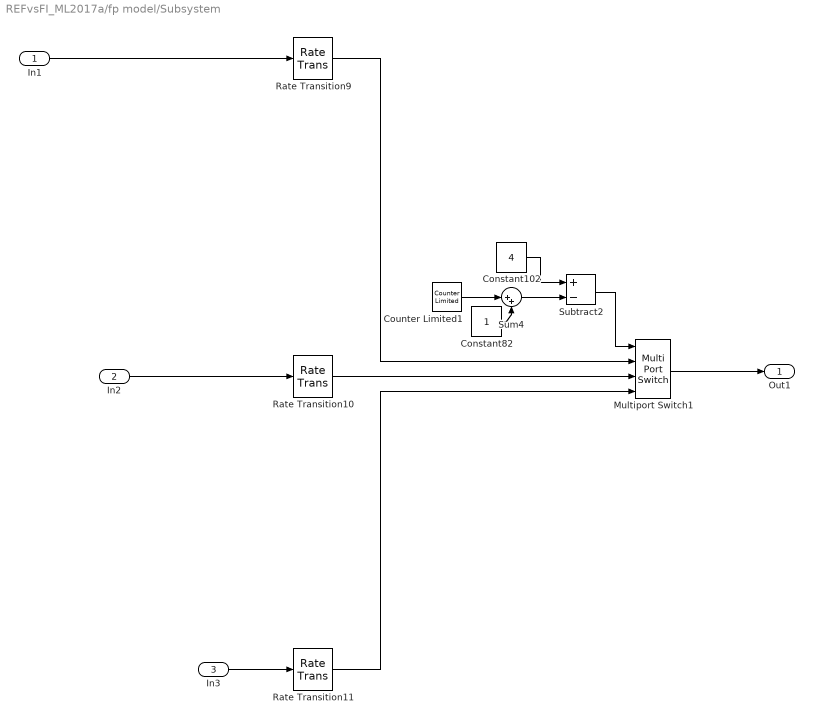
== system REFvsFI_ML2017a/fp model/Subsystem ==
  In1 : Inport
  In2 : Inport  Port=2
  In3 : Inport  Port=3
  Constant102 : Constant  Value=4  OutDataTypeStr=fixdt(0,3,0)
  Constant82 : Constant  OutDataTypeStr=fixdt(0,1,0)
  Counter Limited1 : simulink/Sources/Counter Limited  uplimit=2  tsamp=Ts
  Multiport Switch1 : MultiPortSwitch  OutDataTypeStr=fixdt(1,WL,FLout)  RndMeth=Nearest
  Rate Transition10 : RateTransition  OutPortSampleTime=Ts
  Rate Transition11 : RateTransition  OutPortSampleTime=Ts
  Rate Transition9 : RateTransition  OutPortSampleTime=Ts
  Subtract2 : Sum  Inputs=+-  OutDataTypeStr=fixdt(0,2,0)
  Sum4 : Sum  Inputs=|++  OutDataTypeStr=fixdt(0,2,0)
  Out1 : Outport
  wires:
  Rate Transition11/1 -> Multiport Switch1/4
  Constant82/1 -> Sum4/2
  Subtract2/1 -> Multiport Switch1/1
  Counter Limited1/1 -> Sum4/1
  Sum4/1 -> Subtract2/2
  Constant102/1 -> Subtract2/1
  Rate Transition9/1 -> Multiport Switch1/2
  Rate Transition10/1 -> Multiport Switch1/3
  In2/1 -> Rate Transition10/1
  In1/1 -> Rate Transition9/1
  Multiport Switch1/1 -> Out1/1
  In3/1 -> Rate Transition11/1

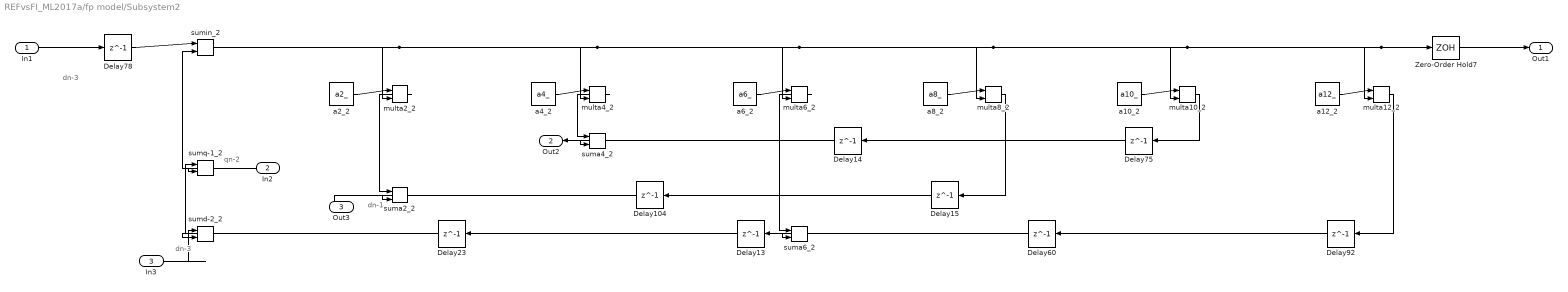
== system REFvsFI_ML2017a/fp model/Subsystem2 ==
  note: dn-1
  note: dn-3
  note: dn-3
  note: qn-2
  In1 : Inport
  In2 : Inport  Port=2
  In3 : Inport  Port=3
  Delay{13..15,23,60,75,78,92,104} (9 alike) : Delay  DelayLength=1  SampleTime=3*Ts
  Zero-Order Hold7 : ZeroOrderHold  SampleTime=3*Ts
  a10_2 : My_FI_Operations/a10_  SystemSampleTime=-1  Latency=0  AutoFrameSizeCalculation=off
  a12_2 : My_FI_Operations/a12_  SystemSampleTime=-1  Latency=0  AutoFrameSizeCalculation=off
  a2_2 : My_FI_Operations/a2_  SystemSampleTime=-1  Latency=0  AutoFrameSizeCalculation=off
  a4_2 : My_FI_Operations/a4_  SystemSampleTime=-1  Latency=0  AutoFrameSizeCalculation=off
  a6_2 : My_FI_Operations/a6_  SystemSampleTime=-1  Latency=0  AutoFrameSizeCalculation=off
  a8_2 : My_FI_Operations/a8_  SystemSampleTime=-1  Latency=0  AutoFrameSizeCalculation=off
  multa10_2 : My_FI_Operations/multa10_  SystemSampleTime=-1  Latency=0  AutoFrameSizeCalculation=off
  multa12_2 : My_FI_Operations/multa12_  SystemSampleTime=-1  Latency=0  AutoFrameSizeCalculation=off
  multa2_2 : My_FI_Operations/multa2_  SystemSampleTime=-1  Latency=0  AutoFrameSizeCalculation=off
  multa4_2 : My_FI_Operations/multa4_  SystemSampleTime=-1  Latency=0  AutoFrameSizeCalculation=off
  multa6_2 : My_FI_Operations/multa6_  SystemSampleTime=-1  Latency=0  AutoFrameSizeCalculation=off
  multa8_2 : My_FI_Operations/multa8_  SystemSampleTime=-1  Latency=0  AutoFrameSizeCalculation=off
  suma2_2 : My_FI_Operations/suma2_  SystemSampleTime=-1  Latency=0  AutoFrameSizeCalculation=off
  suma4_2 : My_FI_Operations/suma4_  SystemSampleTime=-1  Latency=0  AutoFrameSizeCalculation=off
  suma6_2 : My_FI_Operations/suma6_  SystemSampleTime=-1  Latency=0  AutoFrameSizeCalculation=off
  sumd-2_2 : My_FI_Operations/sumd-2_  SystemSampleTime=-1  Latency=0  AutoFrameSizeCalculation=off
  sumin_2 : My_FI_Operations/sumin_  SystemSampleTime=-1  Latency=0  AutoFrameSizeCalculation=off
  sumq-1_2 : My_FI_Operations/sumq-1_  SystemSampleTime=-1  Latency=0  AutoFrameSizeCalculation=off
  Out1 : Outport
  Out2 : Outport  Port=2
  Out3 : Outport  Port=3
  wires:
  sumin_2/1 -> multa2_2/2, multa12_2/2, Zero-Order Hold7/1, multa10_2/2, multa8_2/2, multa6_2/2, multa4_2/2
  In2/1 -> sumq-1_2/2
  a12_2/1 -> multa12_2/1
  Delay78/1 -> sumin_2/1
  sumd-2_2/1 -> sumq-1_2/1
  suma6_2/1 -> Delay13/1
  Zero-Order Hold7/1 -> Out1/1
  sumq-1_2/1 -> sumin_2/2
  Delay15/1 -> Delay104/1
  Delay13/1 -> Delay23/1
  a10_2/1 -> multa10_2/1
  suma4_2/1 -> Out2/1
  In3/1 -> sumd-2_2/1
  multa10_2/1 -> Delay75/1
  multa8_2/1 -> Delay15/1
  multa4_2/1 -> suma4_2/1
  multa2_2/1 -> suma2_2/1
  Delay14/1 -> suma4_2/2
  a2_2/1 -> multa2_2/1
  Delay60/1 -> suma6_2/2
  a8_2/1 -> multa8_2/1
  multa6_2/1 -> suma6_2/1
  Delay75/1 -> Delay14/1
  multa12_2/1 -> Delay92/1
  a4_2/1 -> multa4_2/1
  a6_2/1 -> multa6_2/1
  Delay23/1 -> sumd-2_2/2
  Delay104/1 -> suma2_2/2
  In1/1 -> Delay78/1
  Delay92/1 -> Delay60/1
  suma2_2/1 -> Out3/1

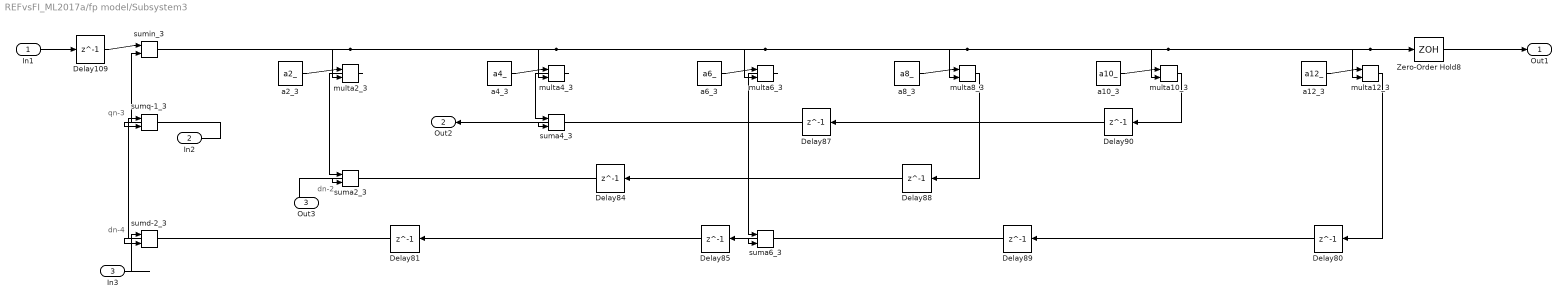
== system REFvsFI_ML2017a/fp model/Subsystem3 ==
  note: dn-2
  note: dn-4
  note: qn-3
  In1 : Inport
  In2 : Inport  Port=2
  In3 : Inport  Port=3
  Delay{80..81,84..85,87..90,109} (9 alike) : Delay  DelayLength=1  SampleTime=3*Ts
  Zero-Order Hold8 : ZeroOrderHold  SampleTime=3*Ts
  a10_3 : My_FI_Operations/a10_  SystemSampleTime=-1  Latency=0  AutoFrameSizeCalculation=off
  a12_3 : My_FI_Operations/a12_  SystemSampleTime=-1  Latency=0  AutoFrameSizeCalculation=off
  a2_3 : My_FI_Operations/a2_  SystemSampleTime=-1  Latency=0  AutoFrameSizeCalculation=off
  a4_3 : My_FI_Operations/a4_  SystemSampleTime=-1  Latency=0  AutoFrameSizeCalculation=off
  a6_3 : My_FI_Operations/a6_  SystemSampleTime=-1  Latency=0  AutoFrameSizeCalculation=off
  a8_3 : My_FI_Operations/a8_  SystemSampleTime=-1  Latency=0  AutoFrameSizeCalculation=off
  multa10_3 : My_FI_Operations/multa10_  SystemSampleTime=-1  Latency=0  AutoFrameSizeCalculation=off
  multa12_3 : My_FI_Operations/multa12_  SystemSampleTime=-1  Latency=0  AutoFrameSizeCalculation=off
  multa2_3 : My_FI_Operations/multa2_  SystemSampleTime=-1  Latency=0  AutoFrameSizeCalculation=off
  multa4_3 : My_FI_Operations/multa4_  SystemSampleTime=-1  Latency=0  AutoFrameSizeCalculation=off
  multa6_3 : My_FI_Operations/multa6_  SystemSampleTime=-1  Latency=0  AutoFrameSizeCalculation=off
  multa8_3 : My_FI_Operations/multa8_  SystemSampleTime=-1  Latency=0  AutoFrameSizeCalculation=off
  suma2_3 : My_FI_Operations/suma2_  SystemSampleTime=-1  Latency=0  AutoFrameSizeCalculation=off
  suma4_3 : My_FI_Operations/suma4_  SystemSampleTime=-1  Latency=0  AutoFrameSizeCalculation=off
  suma6_3 : My_FI_Operations/suma6_  SystemSampleTime=-1  Latency=0  AutoFrameSizeCalculation=off
  sumd-2_3 : My_FI_Operations/sumd-2_  SystemSampleTime=-1  Latency=0  AutoFrameSizeCalculation=off
  sumin_3 : My_FI_Operations/sumin_  SystemSampleTime=-1  Latency=0  AutoFrameSizeCalculation=off
  sumq-1_3 : My_FI_Operations/sumq-1_  SystemSampleTime=-1  Latency=0  AutoFrameSizeCalculation=off
  Out1 : Outport
  Out2 : Outport  Port=2
  Out3 : Outport  Port=3
  wires:
  multa8_3/1 -> Delay88/1
  multa6_3/1 -> suma6_3/1
  Delay84/1 -> suma2_3/2
  sumin_3/1 -> multa2_3/2, multa4_3/2, multa6_3/2, multa8_3/2, multa10_3/2, multa12_3/2, Zero-Order Hold8/1
  multa12_3/1 -> Delay80/1
  In3/1 -> sumd-2_3/1
  suma6_3/1 -> Delay85/1
  Delay85/1 -> Delay81/1
  sumd-2_3/1 -> sumq-1_3/1
  a4_3/1 -> multa4_3/1
  sumq-1_3/1 -> sumin_3/2
  a10_3/1 -> multa10_3/1
  Zero-Order Hold8/1 -> Out1/1
  Delay88/1 -> Delay84/1
  Delay89/1 -> suma6_3/2
  multa2_3/1 -> suma2_3/1
  a12_3/1 -> multa12_3/1
  multa10_3/1 -> Delay90/1
  Delay87/1 -> suma4_3/2
  Delay90/1 -> Delay87/1
  Delay80/1 -> Delay89/1
  a6_3/1 -> multa6_3/1
  a8_3/1 -> multa8_3/1
  a2_3/1 -> multa2_3/1
  multa4_3/1 -> suma4_3/1
  suma2_3/1 -> Out3/1
  In2/1 -> sumq-1_3/2
  suma4_3/1 -> Out2/1
  In1/1 -> Delay109/1
  Delay109/1 -> sumin_3/1
  Delay81/1 -> sumd-2_3/2

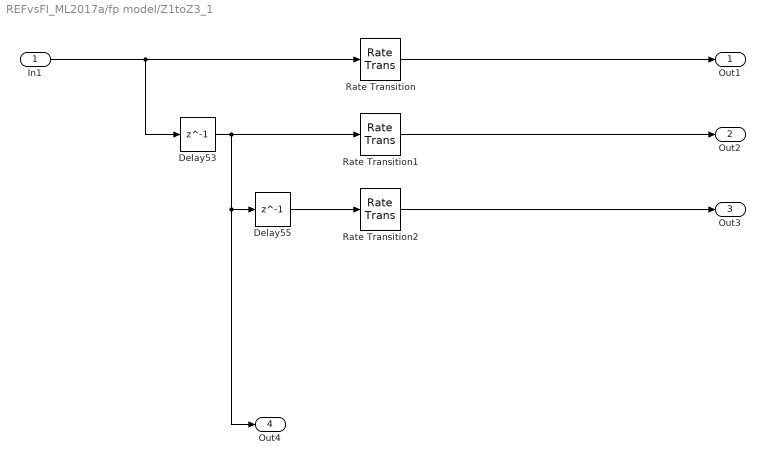
== system REFvsFI_ML2017a/fp model/Z1toZ3_1 ==
  In1 : Inport
  Delay53 : Delay  DelayLength=1  SampleTime=Ts
  Delay55 : Delay  DelayLength=1  SampleTime=Ts
  Rate Transition : RateTransition  OutPortSampleTime=3*Ts
  Rate Transition1 : RateTransition  OutPortSampleTime=3*Ts
  Rate Transition2 : RateTransition  OutPortSampleTime=3*Ts
  Out1 : Outport
  Out2 : Outport  Port=2
  Out3 : Outport  Port=3
  Out4 : Outport  Port=4
  wires:
  Delay53/1 -> Rate Transition1/1, Out4/1, Delay55/1
  Delay55/1 -> Rate Transition2/1
  In1/1 -> Delay53/1, Rate Transition/1
  Rate Transition/1 -> Out1/1
  Rate Transition1/1 -> Out2/1
  Rate Transition2/1 -> Out3/1

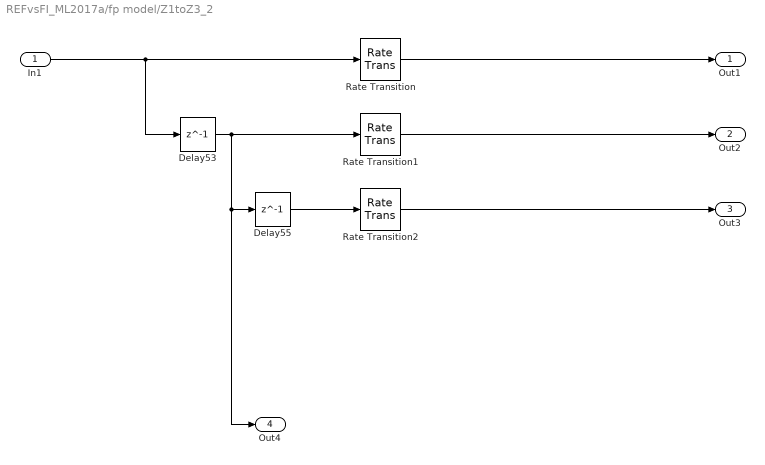
== system REFvsFI_ML2017a/fp model/Z1toZ3_2 ==
  In1 : Inport
  Delay53 : Delay  DelayLength=1  SampleTime=Ts
  Delay55 : Delay  DelayLength=1  SampleTime=Ts
  Rate Transition : RateTransition  OutPortSampleTime=3*Ts
  Rate Transition1 : RateTransition  OutPortSampleTime=3*Ts
  Rate Transition2 : RateTransition  OutPortSampleTime=3*Ts
  Out1 : Outport
  Out2 : Outport  Port=2
  Out3 : Outport  Port=3
  Out4 : Outport  Port=4
  wires:
  Delay53/1 -> Rate Transition1/1, Out4/1, Delay55/1
  Delay55/1 -> Rate Transition2/1
  In1/1 -> Delay53/1, Rate Transition/1
  Rate Transition/1 -> Out1/1
  Rate Transition1/1 -> Out2/1
  Rate Transition2/1 -> Out3/1

== system REFvsFI_ML2017a/fp model/Z1toZ3_3 ==
  In1 : Inport
  Delay53 : Delay  DelayLength=1  SampleTime=Ts
  Delay55 : Delay  DelayLength=1  SampleTime=Ts
  Rate Transition : RateTransition  OutPortSampleTime=3*Ts
  Rate Transition1 : RateTransition  OutPortSampleTime=3*Ts
  Rate Transition2 : RateTransition  OutPortSampleTime=3*Ts
  Out1 : Outport
  Out2 : Outport  Port=2
  Out3 : Outport  Port=3
  Out4 : Outport  Port=4
  wires:
  Delay53/1 -> Rate Transition1/1, Out4/1, Delay55/1
  Delay55/1 -> Rate Transition2/1
  In1/1 -> Delay53/1, Rate Transition/1
  Rate Transition/1 -> Out1/1
  Rate Transition1/1 -> Out2/1
  Rate Transition2/1 -> Out3/1

== system REFvsFI_ML2017a/ref model/multa10_1 ==
  In2 : Inport
  In1 : Inport  Port=2
  Product : Product  OutDataTypeStr=double  RndMeth=Nearest
  Out1 : Outport
  wires:
  Product/1 -> Out1/1
  In2/1 -> Product/2
  In1/1 -> Product/1

== system REFvsFI_ML2017a/ref model/multa10_2 ==
  In2 : Inport
  In1 : Inport  Port=2
  Product : Product  OutDataTypeStr=double  RndMeth=Nearest
  Out1 : Outport
  wires:
  Product/1 -> Out1/1
  In2/1 -> Product/2
  In1/1 -> Product/1

== system REFvsFI_ML2017a/ref model/multa10_3 ==
  In2 : Inport
  In1 : Inport  Port=2
  Product : Product  OutDataTypeStr=double  RndMeth=Nearest
  Out1 : Outport
  wires:
  Product/1 -> Out1/1
  In2/1 -> Product/2
  In1/1 -> Product/1

== system REFvsFI_ML2017a/ref model/multa12_1 ==
  In2 : Inport
  In1 : Inport  Port=2
  Product : Product  OutDataTypeStr=double  RndMeth=Nearest
  Out1 : Outport
  wires:
  Product/1 -> Out1/1
  In1/1 -> Product/1
  In2/1 -> Product/2

== system REFvsFI_ML2017a/ref model/multa12_2 ==
  In2 : Inport
  In1 : Inport  Port=2
  Product : Product  OutDataTypeStr=double  RndMeth=Nearest
  Out1 : Outport
  wires:
  Product/1 -> Out1/1
  In1/1 -> Product/1
  In2/1 -> Product/2

== system REFvsFI_ML2017a/ref model/multa12_3 ==
  In2 : Inport
  In1 : Inport  Port=2
  Product : Product  OutDataTypeStr=double  RndMeth=Nearest
  Out1 : Outport
  wires:
  Product/1 -> Out1/1
  In1/1 -> Product/1
  In2/1 -> Product/2

== system REFvsFI_ML2017a/ref model/multa2_1 ==
  In2 : Inport
  In1 : Inport  Port=2
  Product : Product  OutDataTypeStr=double  RndMeth=Nearest
  Out1 : Outport
  wires:
  Product/1 -> Out1/1
  In1/1 -> Product/1
  In2/1 -> Product/2

== system REFvsFI_ML2017a/ref model/multa2_2 ==
  In2 : Inport
  In1 : Inport  Port=2
  Product : Product  OutDataTypeStr=double  RndMeth=Nearest
  Out1 : Outport
  wires:
  Product/1 -> Out1/1
  In1/1 -> Product/1
  In2/1 -> Product/2

== system REFvsFI_ML2017a/ref model/multa2_3 ==
  In2 : Inport
  In1 : Inport  Port=2
  Product : Product  OutDataTypeStr=double  RndMeth=Nearest
  Out1 : Outport
  wires:
  Product/1 -> Out1/1
  In1/1 -> Product/1
  In2/1 -> Product/2

== system REFvsFI_ML2017a/ref model/multa4_1 ==
  In2 : Inport
  In1 : Inport  Port=2
  Product : Product  OutDataTypeStr=double  RndMeth=Nearest
  Out1 : Outport
  wires:
  In2/1 -> Product/2
  Product/1 -> Out1/1
  In1/1 -> Product/1

== system REFvsFI_ML2017a/ref model/multa4_2 ==
  In2 : Inport
  In1 : Inport  Port=2
  Product : Product  OutDataTypeStr=double  RndMeth=Nearest
  Out1 : Outport
  wires:
  In2/1 -> Product/2
  Product/1 -> Out1/1
  In1/1 -> Product/1

== system REFvsFI_ML2017a/ref model/multa4_3 ==
  In2 : Inport
  In1 : Inport  Port=2
  Product : Product  OutDataTypeStr=double  RndMeth=Nearest
  Out1 : Outport
  wires:
  In2/1 -> Product/2
  Product/1 -> Out1/1
  In1/1 -> Product/1

== system REFvsFI_ML2017a/ref model/multa6_1 ==
  In2 : Inport
  In1 : Inport  Port=2
  Product : Product  OutDataTypeStr=double  RndMeth=Nearest
  Out1 : Outport
  wires:
  Product/1 -> Out1/1
  In2/1 -> Product/2
  In1/1 -> Product/1

== system REFvsFI_ML2017a/ref model/multa6_2 ==
  In2 : Inport
  In1 : Inport  Port=2
  Product : Product  OutDataTypeStr=double  RndMeth=Nearest
  Out1 : Outport
  wires:
  Product/1 -> Out1/1
  In2/1 -> Product/2
  In1/1 -> Product/1

== system REFvsFI_ML2017a/ref model/multa6_3 ==
  In2 : Inport
  In1 : Inport  Port=2
  Product : Product  OutDataTypeStr=double  RndMeth=Nearest
  Out1 : Outport
  wires:
  Product/1 -> Out1/1
  In2/1 -> Product/2
  In1/1 -> Product/1

== system REFvsFI_ML2017a/ref model/multa8_1 ==
  In2 : Inport
  In1 : Inport  Port=2
  Product : Product  OutDataTypeStr=double  RndMeth=Nearest
  Out1 : Outport
  wires:
  Product/1 -> Out1/1
  In2/1 -> Product/2
  In1/1 -> Product/1

== system REFvsFI_ML2017a/ref model/multa8_2 ==
  In2 : Inport
  In1 : Inport  Port=2
  Product : Product  OutDataTypeStr=double  RndMeth=Nearest
  Out1 : Outport
  wires:
  Product/1 -> Out1/1
  In2/1 -> Product/2
  In1/1 -> Product/1

== system REFvsFI_ML2017a/ref model/multa8_3 ==
  In2 : Inport
  In1 : Inport  Port=2
  Product : Product  OutDataTypeStr=double  RndMeth=Nearest
  Out1 : Outport
  wires:
  Product/1 -> Out1/1
  In2/1 -> Product/2
  In1/1 -> Product/1

== system REFvsFI_ML2017a/ref model/multb0_1 ==
  In2 : Inport
  In1 : Inport  Port=2
  Product : Product  OutDataTypeStr=double  RndMeth=Nearest
  Out1 : Outport
  wires:
  In2/1 -> Product/2
  Product/1 -> Out1/1
  In1/1 -> Product/1

== system REFvsFI_ML2017a/ref model/multb0_2 ==
  In2 : Inport
  In1 : Inport  Port=2
  Product : Product  OutDataTypeStr=double  RndMeth=Nearest
  Out1 : Outport
  wires:
  In2/1 -> Product/2
  Product/1 -> Out1/1
  In1/1 -> Product/1

== system REFvsFI_ML2017a/ref model/multb0_3 ==
  In2 : Inport
  In1 : Inport  Port=2
  Product : Product  OutDataTypeStr=double  RndMeth=Nearest
  Out1 : Outport
  wires:
  In2/1 -> Product/2
  Product/1 -> Out1/1
  In1/1 -> Product/1

== system REFvsFI_ML2017a/ref model/multb10_1 ==
  In2 : Inport
  In1 : Inport  Port=2
  Product : Product  OutDataTypeStr=double  RndMeth=Nearest
  Out1 : Outport
  wires:
  Product/1 -> Out1/1
  In1/1 -> Product/1
  In2/1 -> Product/2

== system REFvsFI_ML2017a/ref model/multb10_2 ==
  In2 : Inport
  In1 : Inport  Port=2
  Product : Product  OutDataTypeStr=double  RndMeth=Nearest
  Out1 : Outport
  wires:
  Product/1 -> Out1/1
  In1/1 -> Product/1
  In2/1 -> Product/2

== system REFvsFI_ML2017a/ref model/multb10_3 ==
  In2 : Inport
  In1 : Inport  Port=2
  Product : Product  OutDataTypeStr=double  RndMeth=Nearest
  Out1 : Outport
  wires:
  Product/1 -> Out1/1
  In1/1 -> Product/1
  In2/1 -> Product/2

== system REFvsFI_ML2017a/ref model/multb12_1 ==
  In2 : Inport
  In1 : Inport  Port=2
  Product : Product  OutDataTypeStr=double  RndMeth=Nearest
  Out1 : Outport
  wires:
  Product/1 -> Out1/1
  In1/1 -> Product/1
  In2/1 -> Product/2

== system REFvsFI_ML2017a/ref model/multb12_2 ==
  In2 : Inport
  In1 : Inport  Port=2
  Product : Product  OutDataTypeStr=double  RndMeth=Nearest
  Out1 : Outport
  wires:
  Product/1 -> Out1/1
  In1/1 -> Product/1
  In2/1 -> Product/2

== system REFvsFI_ML2017a/ref model/multb12_3 ==
  In2 : Inport
  In1 : Inport  Port=2
  Product : Product  OutDataTypeStr=double  RndMeth=Nearest
  Out1 : Outport
  wires:
  Product/1 -> Out1/1
  In1/1 -> Product/1
  In2/1 -> Product/2

== system REFvsFI_ML2017a/ref model/multb2_1 ==
  In2 : Inport
  In1 : Inport  Port=2
  Product : Product  OutDataTypeStr=double  RndMeth=Nearest
  Out1 : Outport
  wires:
  In1/1 -> Product/1
  In2/1 -> Product/2
  Product/1 -> Out1/1

== system REFvsFI_ML2017a/ref model/multb2_2 ==
  In2 : Inport
  In1 : Inport  Port=2
  Product : Product  OutDataTypeStr=double  RndMeth=Nearest
  Out1 : Outport
  wires:
  In1/1 -> Product/1
  In2/1 -> Product/2
  Product/1 -> Out1/1

== system REFvsFI_ML2017a/ref model/multb2_3 ==
  In2 : Inport
  In1 : Inport  Port=2
  Product : Product  OutDataTypeStr=double  RndMeth=Nearest
  Out1 : Outport
  wires:
  In1/1 -> Product/1
  In2/1 -> Product/2
  Product/1 -> Out1/1

== system REFvsFI_ML2017a/ref model/multb4_1 ==
  In2 : Inport
  In1 : Inport  Port=2
  Product : Product  OutDataTypeStr=double  RndMeth=Nearest
  Out1 : Outport
  wires:
  In2/1 -> Product/2
  In1/1 -> Product/1
  Product/1 -> Out1/1
